simulink model "Sorrunding"  (R2023b)
settings: Solver=VariableStepAuto  StartTime=0.0  StopTime=10.0  RelTol=1e-3
settings Model: Creator=user  LastModifiedBy=user

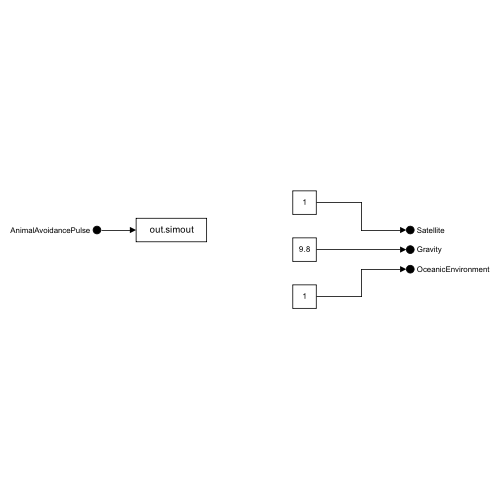
[thumbnail: Simulink's stored preview of the top-level diagram]
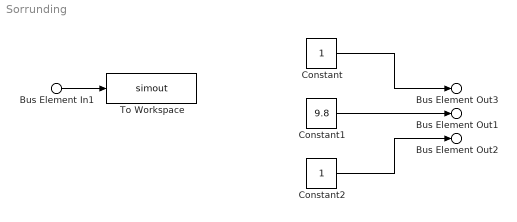
== system Sorrunding ==
  Bus Element In1 : Inport  PortName=AnimalAvoidancePulse
  Constant : Constant
  Constant1 : Constant  Value=9.8
  Constant2 : Constant
  To Workspace : ToWorkspace  VariableName=simout  SampleTime=-1
  Bus Element Out3 : Outport  PortName=Satellite
  Bus Element Out1 : Outport  Port=2  PortName=Gravity
  Bus Element Out2 : Outport  Port=3  PortName=OceanicEnvironment
  wires:
  Bus Element In1/1 -> To Workspace/1
  Constant/1 -> Bus Element Out3/1
  Constant1/1 -> Bus Element Out1/1
  Constant2/1 -> Bus Element Out2/1
